simulink model "nonlinear_simulink_model"  (R2024b)
settings: Solver=FixedStepAuto  StartTime=0.0  StopTime=10.0  FixedStep=1e-4  MaxStep=1e-3  RelTol=1e-3
values from neighbouring files (symbols this model uses):
  G_hov = [ 0 0 0 0 0 0 1 0 ]    [linear_controller_compute_no_integ.m]    (also in new_strategy.m = [1 0 0 0 0 0 0 0])
  G_pos = [ 1 0 0 0 ... (first row only)    [linear_controller_compute_no_integ.m]    (also in new_strategy.m = [1 0 0 0)
  K_att = lqr(sys_red_int, Q, R)    [new_strategy.m]
  K_hor = lqr(sys_hor_int, Q_hor, R_hor)    [new_strategy.m]
  params = [m; Jx; Jy; Jz; c; r; g]    [new_strategy.m]
  X0 = [0;0;3; 0;0;0; 0;0;0; 0;0;0]    [new_strategy.m]
settings Model: Creator=yoonj  LastModifiedBy=yoonj

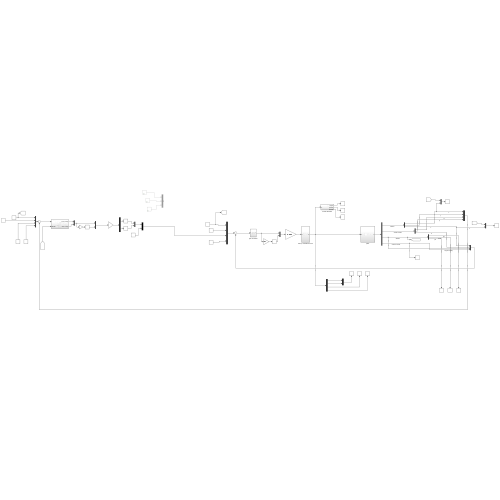
[thumbnail: Simulink's stored preview of the top-level diagram]
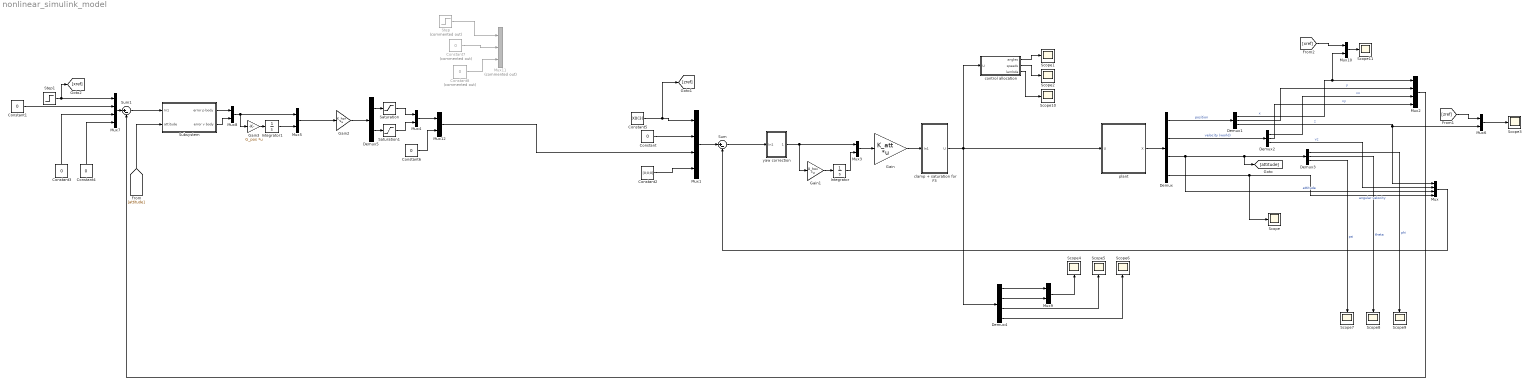
== system nonlinear_simulink_model ==
  Constant{,1,3..4,6} (5 alike) : Constant  Value=0
  Constant2 : Constant  Value=[0;0;0]  VectorParams1D=off
  Constant5 : Constant  Value=X0(3)
  Constant7 : Constant  Commented=on  Value=0
  Constant8 : Constant  Commented=on  Value=0
  Demux : Demux
  Demux1 : Demux  Outputs=3
  Demux2 : Demux  Outputs=3
  Demux3 : Demux  Outputs=3
  Demux4 : Demux
  Demux5 : Demux  Outputs=2
  Gain : Gain  Gain=K_att  Multiplication=Matrix(K*u)
  Gain1 : Gain  Gain=G_hov  Multiplication=Matrix(K*u)
  Gain2 : Gain  Gain=K_hor  Multiplication=Matrix(K*u)
  Gain3 : Gain  Gain=G_pos  Multiplication=Matrix(K*u)
  Integrator : Integrator  InitialCondition=X0(3)
  Integrator1 : Integrator  InitialCondition=[X0(1); X0(2)]  UpperSaturationLimit=0.4  LowerSaturationLimit=-0.4
  Mux{,1..2,7} (4 alike) : Mux
  Mux{3..6,8..10,12} (8 alike) : Mux  Inputs=2
  Mux11 : Mux  Commented=on  Inputs=3
  Saturation : Saturate  UpperLimit=0.2  LowerLimit=-0.2
  Saturation1 : Saturate  UpperLimit=0.2  LowerLimit=-0.2
  Scope{,1..11} (12 alike) : Scope
  Step : Step  Commented=on  After=0.8  SampleTime=0
  Step1 : Step  After=0.1  SampleTime=0
  Subsystem : Subsystem
  Sum : Sum  Inputs=|+-
  Sum1 : Sum  Inputs=|+-
  clamp + saturation for F3 : Subsystem
  control allocation : Subsystem
  plant : Subsystem
  yaw correction : Subsystem
  wires:
  Demux/1 -> Demux1/1  "position"
  plant/1(X) -> Demux/1
  Demux/2 -> Demux2/1  "velocity (world)"
  Demux1/3 -> Mux6/2, Mux/1  "z"
  Demux2/3 -> Mux/2  "vz"
  Demux/3 -> Mux/3, Demux3/1, [attitude]  "attitude"
  Demux/4 -> Scope/1, Mux/4  "angular velocity"
  Mux/1 -> Sum/2
  Mux1/1 -> Sum/1
  Gain/1 -> clamp + saturation for F3/1(In1)
  clamp + saturation for F3/1(U) -> plant/1(U), control allocation/1(U), Demux4/1
  Constant/1 -> Mux1/2
  Constant2/1 -> Mux1/4
  Mux3/1 -> Gain/1
  Gain1/1 -> Integrator/1
  Integrator/1 -> Mux3/2
  Mux5/1 -> Gain2/1
  Mux7/1 -> Sum1/1
  Step1/1 -> [xref], Mux7/1
  Constant1/1 -> Mux7/2
  Constant3/1 -> Mux7/3
  Constant4/1 -> Mux7/4
  Gain3/1 -> Integrator1/1
  Integrator1/1 -> Mux5/2
  Sum/1 -> yaw correction/1(In1)
  yaw correction/1(Out1) -> Gain1/1, Mux3/1
  Mux8/1 -> Gain3/1, Mux5/1
  Sum1/1 -> Subsystem/1(In1)
  Subsystem/1(error p body) -> Mux8/1
  Subsystem/2(error v body) -> Mux8/2
  Demux1/1 -> Mux10/2, Mux2/1  "x"
  Demux1/2 -> Mux2/2  "y"
  Demux2/1 -> Mux2/3  "vx"
  Demux2/2 -> Mux2/4  "vy"
  control allocation/1(angles) -> Scope1/1
  control allocation/2(speeds) -> Scope2/1
  Mux6/1 -> Scope3/1
  Demux4/1 -> Mux9/1
  Demux4/2 -> Mux9/2
  Mux9/1 -> Scope4/1
  Demux4/3 -> Scope5/1
  Demux4/4 -> Scope6/1
  Demux3/3 -> Scope7/1  "psi"
  Demux3/2 -> Scope8/1  "theta"
  Demux3/1 -> Scope9/1  "phi"
  [attitude] -> Subsystem/2(attitude)
  [zref] -> Mux6/1
  Constant5/1 -> [zref], Mux1/1
  Mux10/1 -> Scope11/1
  [xref] -> Mux10/1
  Step/1 -> Mux11/1
  Constant7/1 -> Mux11/2
  Constant8/1 -> Mux11/3
  control allocation/3(lambda) -> Scope10/1
  Gain2/1 -> Demux5/1
  Demux5/1 -> Saturation/1
  Demux5/2 -> Saturation1/1
  Saturation/1 -> Mux4/1
  Saturation1/1 -> Mux4/2
  Mux4/1 -> Mux12/1
  Constant6/1 -> Mux12/2
  Mux12/1 -> Mux1/3
  Mux2/1 -> Sum1/2

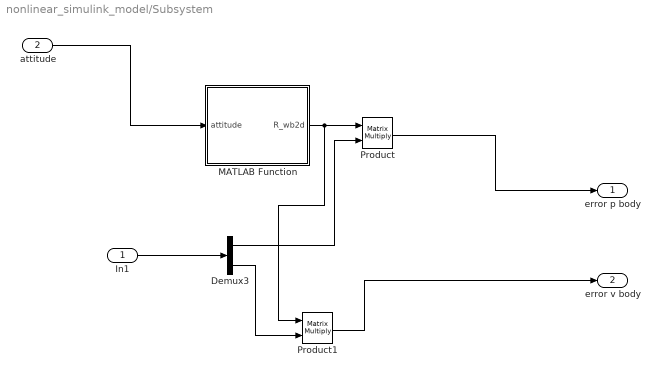
== system nonlinear_simulink_model/Subsystem ==
  In1 : Inport
  attitude : Inport  Port=2
  Demux3 : Demux  Outputs=2
  MATLAB Function : MATLAB Function  TreatAsAtomicUnit=on
  Product : Product  Multiplication=Matrix(*)
  Product1 : Product  Multiplication=Matrix(*)
  error p body : Outport
  error v body : Outport  Port=2
  wires:
  Demux3/1 -> Product/2
  MATLAB Function/1(R_wb2d) -> Product1/1, Product/1
  In1/1 -> Demux3/1
  Product1/1 -> error v body/1
  Demux3/2 -> Product1/2
  Product/1 -> error p body/1
  attitude/1 -> MATLAB Function/1(attitude)

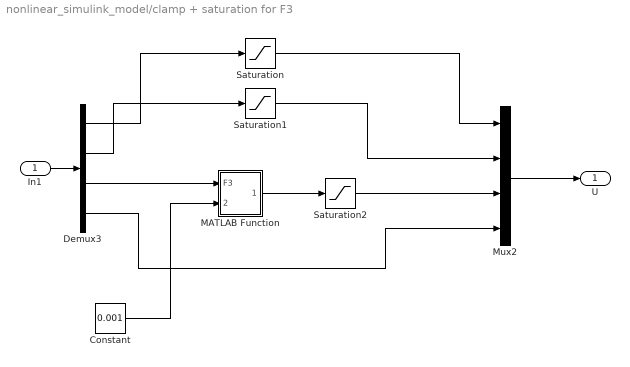
== system nonlinear_simulink_model/clamp + saturation for F3 ==
  In1 : Inport
  Constant : Constant  Value=0.001
  Demux3 : Demux
  MATLAB Function : MATLAB Function  TreatAsAtomicUnit=on
  Mux2 : Mux
  Saturation : Saturate  UpperLimit=3.407  LowerLimit=-3.407
  Saturation1 : Saturate  UpperLimit=3.407  LowerLimit=-3.407
  Saturation2 : Saturate  UpperLimit=19.62  LowerLimit=-19.62
  U : Outport
  wires:
  In1/1 -> Demux3/1
  Demux3/3 -> MATLAB Function/1(F3)
  Demux3/4 -> Mux2/4
  Constant/1 -> MATLAB Function/2(threshold)
  Mux2/1 -> U/1
  Demux3/1 -> Saturation/1
  Saturation/1 -> Mux2/1
  Demux3/2 -> Saturation1/1
  Saturation1/1 -> Mux2/2
  MATLAB Function/1(F3_safe) -> Saturation2/1
  Saturation2/1 -> Mux2/3

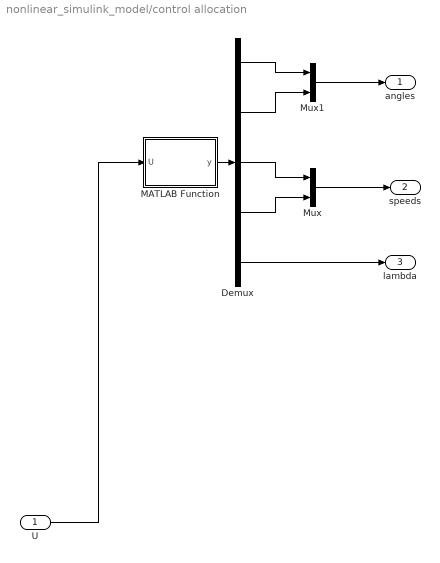
== system nonlinear_simulink_model/control allocation ==
  U : Inport
  Demux : Demux  Outputs=5
  MATLAB Function : MATLAB Function  TreatAsAtomicUnit=on
  Mux : Mux  Inputs=2
  Mux1 : Mux  Inputs=2
  angles : Outport
  speeds : Outport  Port=2
  lambda : Outport  Port=3
  wires:
  U/1 -> MATLAB Function/1(U)
  MATLAB Function/1(y) -> Demux/1
  Demux/5 -> lambda/1
  Demux/3 -> Mux/1
  Demux/4 -> Mux/2
  Mux/1 -> speeds/1
  Mux1/1 -> angles/1
  Demux/1 -> Mux1/1
  Demux/2 -> Mux1/2

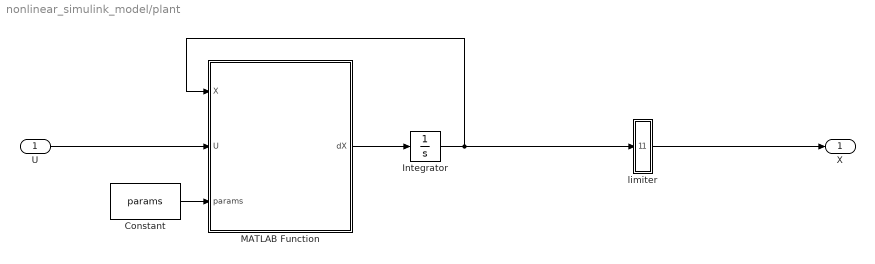
== system nonlinear_simulink_model/plant ==
  U : Inport
  Constant : Constant  Value=params  VectorParams1D=off
  Integrator : Integrator  InitialCondition=X0
  MATLAB Function : MATLAB Function  TreatAsAtomicUnit=on
  limiter : Subsystem
  X : Outport
  wires:
  MATLAB Function/1(dX) -> Integrator/1
  Constant/1 -> MATLAB Function/3(params)
  Integrator/1 -> limiter/1(In1), MATLAB Function/1(X)
  U/1 -> MATLAB Function/2(U)
  limiter/1(Out1) -> X/1

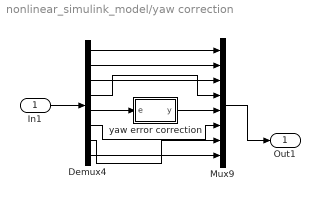
== system nonlinear_simulink_model/yaw correction ==
  In1 : Inport
  Demux4 : Demux  Outputs=8
  Mux9 : Mux  Inputs=8
  yaw error correction : MATLAB Function  TreatAsAtomicUnit=on
  Out1 : Outport
  wires:
  Demux4/5 -> yaw error correction/1(e)
  Demux4/4 -> Mux9/4
  Demux4/6 -> Mux9/6
  Demux4/3 -> Mux9/3
  yaw error correction/1(y) -> Mux9/5
  Demux4/8 -> Mux9/8
  Demux4/1 -> Mux9/1
  Demux4/7 -> Mux9/7
  Demux4/2 -> Mux9/2
  In1/1 -> Demux4/1
  Mux9/1 -> Out1/1

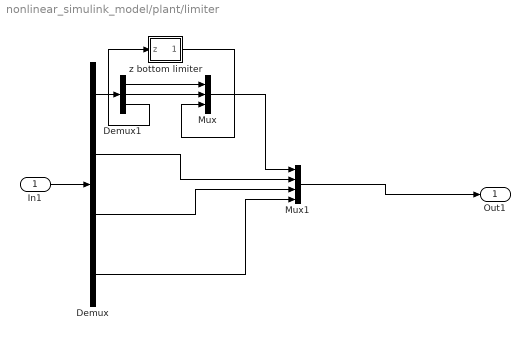
== system nonlinear_simulink_model/plant/limiter ==
  In1 : Inport
  Demux : Demux
  Demux1 : Demux  Outputs=3
  Mux : Mux  Inputs=3
  Mux1 : Mux
  z bottom limiter : MATLAB Function  TreatAsAtomicUnit=on
  Out1 : Outport
  wires:
  z bottom limiter/1(z_true) -> Mux/3
  Demux/2 -> Mux1/2
  Demux1/3 -> z bottom limiter/1(z)
  Demux1/1 -> Mux/1
  Mux/1 -> Mux1/1
  Demux/3 -> Mux1/3
  Demux1/2 -> Mux/2
  Demux/4 -> Mux1/4
  Demux/1 -> Demux1/1
  Mux1/1 -> Out1/1
  In1/1 -> Demux/1

== matlab function nonlinear_simulink_model/plant/MATLAB Function ==
  data: X input; dX output; U input; params input
function dX = rocket_eom(X, U, params)
% ROCKET_EOM  Equations of motion for VTOL rocket (Tait-Bryan ZYX)
%
% State vector X (12x1):
%   X(1)  = x       [m]       inertial position
%   X(2)  = y       [m]
%   X(3)  = z       [m]
%   X(4)  = vx      [m/s]     inertial velocity
%   X(5)  = vy      [m/s]
%   X(6)  = vz      [m/s]
%   X(7)  = phi     [rad]     roll
%   X(8)  = theta   [rad]     pitch
%   X(9)  = psi     [rad]     yaw
%   X(10) = wx      [rad/s]   body angular rates
%   X(11) = wy      [rad/s]
%   X(12) = wz      [rad/s]
%
% Input vector U (4x1):
%   U(1) = F1       [N]       thrust (main engine or gimbal)
%   U(2) = F2       [N]
%   U(3) = F3       [N]
%   U(4) = Mz       [Nm]      yaw moment

% --- Unpack states ---
% vx = X(4); vy = X(5); vz = X(6);  % not needed explicitly below
phi   = X(7);
theta = X(8);
psi   = X(9);
wx    = X(10);
wy    = X(11);
wz    = X(12);

% --- Unpack inputs ---
F1 = U(1);
F2 = U(2);
F3 = U(3);
Mz = U(4);

% --- Parameters (edit as needed) ---
m = params(1);
Jx = params(2);
Jy = params(3);
Jz = params(4);
c = params(5);
r = params(6);
g = params(7);
% --- Precompute trig ---
sphi = sin(phi);   cphi = cos(phi);
sth  = sin(theta); cth  = cos(theta); tth = tan(theta);
spsi = sin(psi);   cpsi = cos(psi);

% --- Shared factor from your symbolic output ---
k = (Mz/(F3*c) - 2);

% --- Position derivatives (= velocities) ---
dx = X(4);
dy = X(5);
dz = X(6);

% --- Velocity derivatives (forces / m) ---
dvx = -(F3*k*(sphi*spsi + cphi*cpsi*sth) ...
       - F2*k*(cphi*spsi - cpsi*sphi*sth) ...
       + F1*cpsi*cth*k) / m;

dvy = -(F2*k*(cphi*cpsi + sphi*spsi*sth) ...
       - F3*k*(cpsi*sphi - cphi*spsi*sth) ...
       + F1*cth*spsi*k) / m;

dvz = -g - (F3*cphi*cth*k ...
           - F1*sth*k ...
           + F2*cth*sphi*k) / m;

% --- Euler angle derivatives (kinematics) ---
dphi   = wx + wz*cphi*tth + wy*sphi*tth;
dtheta =      wy*cphi     - wz*sphi;
dpsi   =     (wz*cphi + wy*sphi) / cth;

% --- Angular rate derivatives (Euler's equations) ---
dwx = (F2*r + Jy*wy*wz - Jz*wy*wz) / Jx;
dwy = -(F1*r + Jx*wx*wz - Jz*wx*wz) / Jy;
dwz = (Mz + Jx*wx*wy - Jy*wx*wy) / Jz;

% --- Assemble output ---
if (X(3) > 0 || dvz > 0)
    % return all derivs
    dX = [dx; dy; dz; dvx; dvy; dvz; dphi; dtheta; dpsi; dwx; dwy; dwz];
else
    dX = [0; 0; 0; 0; 0; 0; dphi; dtheta; dpsi; dwx; dwy; dwz];
end

== matlab function nonlinear_simulink_model/yaw correction/yaw error correction ==
  data: e input; y output
function y = fcn(e)

    if( e > pi )
        e = e - 2* pi; 
    end

    y = e;
end

== matlab function nonlinear_simulink_model/Subsystem/MATLAB Function ==
  data: attitude input; R_wb2d output
function R_wb2d = fcn(attitude)

u = attitude(3);

R_wb2d = [ cos(u), sin(u);
           -sin(u), cos(u)];

end

== matlab function nonlinear_simulink_model/control allocation/MATLAB Function ==
  data: U input; y output
function y = fcn(U)
F1 = U(1);
F2 = U(2);
F3 = U(3);
Mz = U(4);
Kt = 0.021;
c = 0.05;

F_norm = sqrt(F1^2 + F2^2 + F3^2);

alpha_1 = asin((F2/F_norm));

alpha_2 = acos( F3/sqrt(F1^2 + F3^2));

omega_1 = sqrt( F_norm / Kt);

lambda = 1 - (Mz / (c * F3));

F_2norm = lambda * F_norm; 

omega_2 = sqrt( abs(F_2norm) / Kt);



y = [alpha_1; alpha_2; omega_1; omega_2; lambda];

end

== matlab function nonlinear_simulink_model/plant/limiter/z bottom limiter ==
  data: z input; z_true output
function z_true = fcn(z)
if (z < 0)
    z_true = 0;
else
    z_true = z;
end

== matlab function nonlinear_simulink_model/clamp + saturation for F3/MATLAB Function ==
  data: F3 input; F3_safe output; threshold input
function F3_safe = clamp_F3(F3, threshold)
% Prevents F3 passing through zero to avoid singularities
% threshold: the deadzone boundary (e.g. 0.001)

if F3 >= 0 && F3 < threshold
    F3_safe = threshold;
elseif F3 < 0 && F3 > -threshold
    F3_safe = -threshold;
else
    F3_safe = F3;
end

end
